simulink model "MatlabSystemObjectModels_v2"  (R2020b)
settings: Solver=VariableStepAuto  StartTime=0.0  StopTime=5  RelTol=1e-3
values from neighbouring files (symbols this model uses):
  Ts = 1/Fs    [MainSimulink.m]
  W0 = FundamentalFreq*2*pi    [MainSimulink.m]    (also in Sim_AddBranch.m = F0*2*pi)
undefined symbols (not defined in the file or in its folder): DevicePara, PowerFlow, Wbase
libraries: powerlib x12, simplex_lib x4
settings Model: Creator=admin_user  LastModifiedBy=admin_user

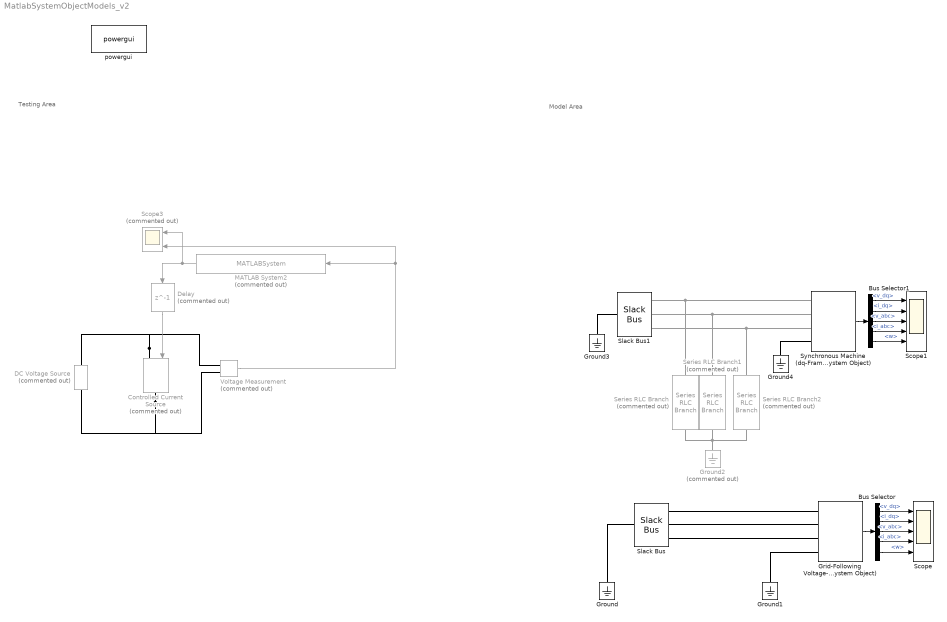
== system MatlabSystemObjectModels_v2 ==
  note: Model Area
  note: Testing Area
  Bus Selector : BusSelector  OutputSignals=v_dq,i_dq,v_abc,i_abc,w
  Bus Selector1 : BusSelector  OutputSignals=v_dq,i_dq,v_abc,i_abc,w
  Controlled Current Source : powerlib/Electrical Sources/Controlled Current Source  Commented=on  Initialize=off  Source_Type=DC  Amplitude=0  Phase=0  Frequency=0  Measurements=None
  DC Voltage Source : powerlib/Electrical Sources/DC Voltage Source  Commented=on  Amplitude=1  Measurements=None
  Delay : Delay  Commented=on  DelayLength=1  InitialCondition=0
  Grid-Following Voltage-Source Inverter (dq-Frame System Object) : simplex_lib/Grid-Following Voltage-Source Inverter (dq-Frame System Object)  Sbase=Sbase  Vbase=Vbase  Wbase=Wbase  Ts=Ts  DeviceType=10  DevicePara=DevicePara{4}  PowerFlow=PowerFlow{4}  x0=[0;0;0;0;2.5;0;0;W0;0]  OtherInputs=[0; 1]
      settings: SourceProductName=Simplex
  Ground{,1,3..4} (4 alike) : powerlib/Elements/Ground  LConnTagsString=a
  Ground2 : powerlib/Elements/Ground  Commented=on  LConnTagsString=a
  MATLAB System2 : MATLABSystem  Commented=on  System=Class_Model_Inductor  DeviceType=90  Para=1  PowerFlow=[0,0,0,0,0]  Ts=Ts  x0=0  SimulateUsing=Code generation
      mask Type: Class_Model_Inductor
      mask Display:
      | disp('Class_Model_Inductor');
      | port_label('input',1,'u');
      | port_label('output',1,'y');
  Scope : Scope  NumInputPorts=5
  Scope1 : Scope  NumInputPorts=5
  Scope3 : Scope  Commented=on  NumInputPorts=2
  Series RLC Branch : powerlib/Elements/Series RLC Branch  Commented=on  LConnTagsString=__new0  RConnTagsString=__new0  BranchType=R  Resistance=1  Inductance=1e-3  SetiL0=off  InitialCurrent=0  Capacitance=1e-6  Setx0=off  InitialVoltage=0  Measurements=None
  Series RLC Branch1 : powerlib/Elements/Series RLC Branch  Commented=on  LConnTagsString=__new0  RConnTagsString=__new0  BranchType=R  Resistance=1  Inductance=1e-3  SetiL0=off  InitialCurrent=0  Capacitance=1e-6  Setx0=off  InitialVoltage=0  Measurements=None
  Series RLC Branch2 : powerlib/Elements/Series RLC Branch  Commented=on  LConnTagsString=__new0  RConnTagsString=__new0  BranchType=R  Resistance=1  Inductance=1e-3  SetiL0=off  InitialCurrent=0  Capacitance=1e-6  Setx0=off  InitialVoltage=0  Measurements=None
  Slack Bus : simplex_lib/Slack Bus  vd=1  vq=0  v0=0  w=1  theta0=0  Vbase=Vbase  Wbase=Wbase
      settings: SourceProductName=Simplex
  Slack Bus1 : simplex_lib/Slack Bus  vd=0.995  vq=0  v0=0  w=1  theta0=0  Vbase=Vbase  Wbase=Wbase
      settings: SourceProductName=Simplex
  Synchronous Machine (dq-Frame System Object) : simplex_lib/Synchronous Machine (dq-Frame System Object)  Sbase=Sbase  Vbase=Vbase  Wbase=Wbase  Ts=Ts  DeviceType=0  DevicePara=DevicePara{1}  PowerFlow=PowerFlow{1}  x0=[0;0;Wbase;0]  OtherInputs=[-10.89/Wbase;0]
      settings: SourceProductName=Simplex
  Voltage Measurement : powerlib/Measurements/Voltage Measurement  Commented=on  PhasorSimulation=off  OutputType=Magnitude  PSBequivalent=0
  powergui : powerlib/powergui  Priority=1  SimulationMode=Discrete  SampleTime=Ts  frequency=60  Iterations=50  frequencyindice=0  Pbase=100e6  ErrMax=1e-4  UnitsV=kV  UnitsW=MW  buscounter=0  FunctionMessages=off  echomessages=off  EnableUseOfTLC=off  CurrentSourceSwitches=off  DisableSnubberDevices=off  DisableRonSwitches=off  DisableVfSwitches=off  DisplayEquations=off  AutomaticDiscreteSolvers=off  SolverType=Tustin  Interpol=off  ExternalGateDelay=off  methode=off  Ts=100  x0status=blocks  SPID=off  SwTol=0  HookPort=off  NonlinearTolerance=1e-4  nMaxIteration=100  ContinueOnMaxIteration=off  RestoreLinks=warning  ResistiveCurrentMeasurement=off  Frange=[0:2:500]  Ylog=off  Xlog=on  ShowGrid=off  save=off  variable=ZData  structure=0  ZoomFFT=off  StartTime=0.0  cycles=1  DisplayStyle=1  fundamental=60  FreqAxis=off  MaxFrequency=1000  frequencyindicesteady=1  RmsSteady=1  display=off
  wires:
  MATLAB System2/1 -> Delay/1, Scope3/1
  Delay/1 -> Controlled Current Source/1
  Voltage Measurement/1 -> Scope3/2, MATLAB System2/1
  Grid-Following Voltage-Source Inverter (dq-Frame System Object)/1 -> Bus Selector/1
  Synchronous Machine (dq-Frame System Object)/1 -> Bus Selector1/1
  Bus Selector/1 -> Scope/1  "<v_dq>"
  Bus Selector/2 -> Scope/2  "<i_dq>"
  Bus Selector/3 -> Scope/3  "<v_abc>"
  Bus Selector/4 -> Scope/4  "<i_abc>"
  Bus Selector/5 -> Scope/5  "<w>"
  Bus Selector1/1 -> Scope1/1  "<v_dq>"
  Bus Selector1/2 -> Scope1/2  "<i_dq>"
  Bus Selector1/3 -> Scope1/3  "<v_abc>"
  Bus Selector1/4 -> Scope1/4  "<i_abc>"
  Bus Selector1/5 -> Scope1/5  "<w>"
  connections:
  Controlled Current Source/RConn1 -- Voltage Measurement/LConn2 -- DC Voltage Source/LConn1
  Controlled Current Source/LConn1 -- Voltage Measurement/LConn1 -- DC Voltage Source/RConn1
  Grid-Following Voltage-Source Inverter (dq-Frame System Object)/LConn1 -- Slack Bus/RConn1
  Grid-Following Voltage-Source Inverter (dq-Frame System Object)/LConn2 -- Slack Bus/RConn2
  Grid-Following Voltage-Source Inverter (dq-Frame System Object)/LConn3 -- Slack Bus/RConn3
  Grid-Following Voltage-Source Inverter (dq-Frame System Object)/LConn4 -- Ground1/LConn1
  Slack Bus/LConn1 -- Ground/LConn1
  Series RLC Branch/RConn1 -- Ground2/LConn1 -- Series RLC Branch2/RConn1 -- Series RLC Branch1/RConn1
  Slack Bus1/LConn1 -- Ground3/LConn1
  Series RLC Branch/LConn1 -- Synchronous Machine (dq-Frame System Object)/LConn1 -- Slack Bus1/RConn1
  Series RLC Branch1/LConn1 -- Synchronous Machine (dq-Frame System Object)/LConn2 -- Slack Bus1/RConn2
  Series RLC Branch2/LConn1 -- Synchronous Machine (dq-Frame System Object)/LConn3 -- Slack Bus1/RConn3
  Synchronous Machine (dq-Frame System Object)/LConn4 -- Ground4/LConn1
